simulink model "PWMSimu"  (R2018a)
settings: Solver=VariableStepAuto  StartTime=0.0  StopTime=10.0  RelTol=1e-3
settings Model: Creator=shahb  LastModifiedBy=shahb

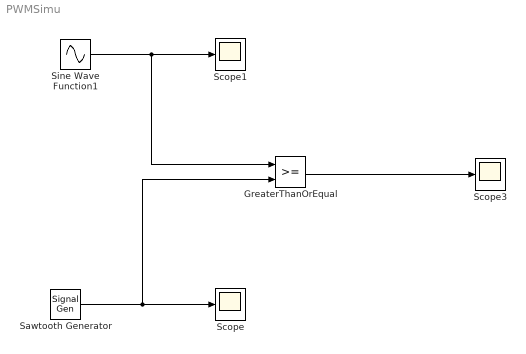
== system PWMSimu ==
  GreaterThanOrEqual : RelationalOperator  OutDataTypeStr=boolean  RndMeth=Simplest
  Sawtooth Generator : SignalGenerator  WaveForm=sawtooth  Amplitude=5  Frequency=5  Units=rad/sec
  Scope : Scope
  Scope1 : Scope
  Scope3 : Scope
  Sine Wave Function1 : Sin  SampleTime=0
  wires:
  Sine Wave Function1/1 -> GreaterThanOrEqual/1, Scope1/1
  Sawtooth Generator/1 -> GreaterThanOrEqual/2, Scope/1
  GreaterThanOrEqual/1 -> Scope3/1
